simulink model "TrayectoriaReal"  (R2018a)
settings: Solver=ode45  StartTime=0.0  StopTime=Tfin2  RelTol=1e-3  EnableMultiTasking=on
values from neighbouring files (symbols this model uses):
  dyn = [dh dyn]    [trabajoRob.m]
  dyne = (ones(6,20)+err).*dyn    [trabajoRob.m]
  g = [0 0 -9.81]    [trabajoRob.m]
  Qt2 = [[1:length(Qt2)]'*Ts2,Qt2]    [trabajoRob.m]    (also in trayectoria.m = [[0:length(trayq)-1]'*Ts2 trayq])
  Tfin = 25    [trabajoRob.m]
  Ts = Tfin/(puntos-1)    (= 0.0501002004008)    [trabajoRob.m]
  Ts2 = 0.01    [trabajoRob.m]    (also in trayectoria.m)
libraries: HEMERO x2, peGeneralControl x2
settings Model: ExtModeTrigMode=oneshot  ExtModeArmWhenConnect=off  Creator=Pablo Linares  LastModifiedBy=Pablo Linares
settings DataIOCC: SaveFormat=Array  SignalLoggingSaveFormat=ModelDataLogs
settings OptimizationCC: BlockReduction=off  BooleanDataType=off
settings DebuggingCC: SaveWithParameterizedLinksMsg=none  UnderspecifiedInitializationDetection=Classic  MergeDetectMultiDrivingBlocksExec=none  SignalResolutionControl=TryResolveAllWithWarning  MultiTaskDSMMsg=warning  MultiTaskCondExecSysMsg=none
settings HardwareCC: TargetUnknown=on
settings ModelReferenceCC: PropagateSignalLabelsOutOfModel=off
settings GRTTargetCC: TargetLangStandard=C89/C90 (ANSI)  CombineOutputUpdateFcns=off  GRTInterface=on

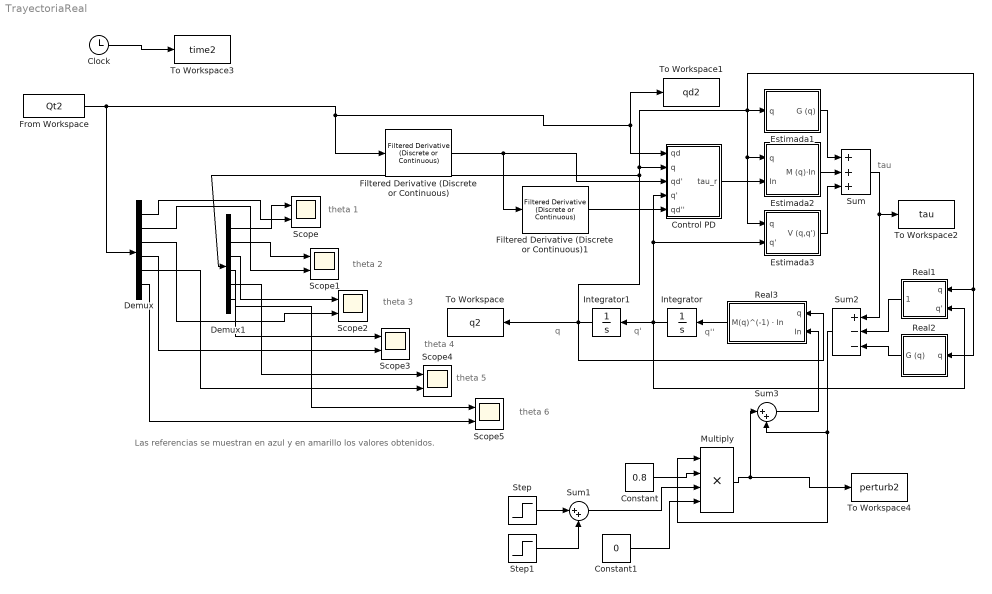
== system TrayectoriaReal ==
  note: Las referencias se muestran en azul y en amarillo los valores obtenidos.
  note: theta 6
  note: theta 5
  note: theta 4
  note: theta 3
  note: theta 2
  note: theta 1
  note: tau
  note: q
  note: q'
  note: q''
  Clock : Clock
  Constant : Constant  Value=0.8
  Constant1 : Constant  Value=0
  Control PD : Subsystem  mask(Controlador PD){Kp=[1 0 0 0 0 0;0 1 0 0 0 0; 0 0 1 0 0 0; 0 0 0 1 0 0; 0 0 0 0 1 0; 0 0 0 0 0 1]*986.96, Kv=[1 0 0 0 0 0;0 1 0 0 0 0; 0 0 1 0 0 0; 0 0 0 1 0 0; 0 0 0 0 1 0; 0 0 0 0 0 1]*62.83}
      mask prompts: Kp "Introduzca la matriz Kp:"; Kv "Introduzca la matriz Kv:"
      mask help: Calcula el par tau_r correspondiente a la técnica del par computado usando un controlador PD.
  Demux : Demux  Outputs=6
  Demux1 : Demux  Outputs=6
  Estimada1 : Subsystem  mask(Término gravitatorio){dyn=dyne, grav=g}
      mask prompts: dyn "Matriz de parámetros cinemáticos y dinámicos:"; grav "Vector aceleración de la gravedad:"
      mask help: Este bloque calcula el par correspondiente al término gravitatorio.
  Estimada2 : Subsystem  mask(Término asociado a la matriz de masas){dyn=dyne}
      mask prompts: dyn "Matriz de parámetros cinemáticos y dinámicos:"
      mask help: Este bloque calcula el par correspondiente al término en el que aparece la matriz de masas.
  Estimada3 : Subsystem  mask(Términos centrífugos y de Coriolis){dyn=dyne}
      mask prompts: dyn "Matriz de parámetros cinemáticos y dinámicos:"
      mask help: Este bloque calcula el par correspondiente a los términos centrífugos y de Coriolis.
  Filtered Derivative (Discrete or Continuous) : peGeneralControl/Filtered Derivative (Discrete or Continuous)  K=1  T=0.01  B=inf  A=-inf  minRatio=10  Ts=Ts
  Filtered Derivative (Discrete or Continuous)1 : peGeneralControl/Filtered Derivative (Discrete or Continuous)  K=1  T=0.01  B=inf  A=-inf  minRatio=10  Ts=Ts
  From Workspace : FromWorkspace  VariableName=Qt2  SampleTime=Ts2
  Integrator : Integrator  InitialCondition=[0;0;0;0;0;0]
  Integrator1 : Integrator  InitialCondition=Qt2(1,2:7)'
  Multiply : Product  Inputs=4
  Real1 : Subsystem  mask(Términos centrífugos y de Coriolis){dyn=dyn}
      mask prompts: dyn "Matriz de parámetros cinemáticos y dinámicos:"
      mask help: Este bloque calcula el par correspondiente a los términos centrífugos y de Coriolis.
  Real2 : Subsystem  mask(Término gravitatorio){dyn=dyn, grav=g}
      mask prompts: dyn "Matriz de parámetros cinemáticos y dinámicos:"; grav "Vector aceleración de la gravedad:"
      mask help: Este bloque calcula el par correspondiente al término gravitatorio.
  Real3 : Subsystem  mask(Inversa de la matriz de masas){dyn=dyn}
      mask prompts: dyn "Matriz de parámetros cinemáticos y dinámicos:"
      mask help: Este bloque calcula el producto de la inversa de la matriz de masas por el vector columna In que se le pasa como entrada.
  Scope{,1..5} (6 alike) : Scope  NumInputPorts=2
  Step : Step  Time=Tfin*0.5  SampleTime=0
  Step1 : Step  Time=Tfin*0.6  After=-1  SampleTime=0
  Sum : Sum  Inputs=+++  SaturateOnIntegerOverflow=on  InputSameDT=on  OutDataTypeStr=Inherit: Same as first input
  Sum1 : Sum  Inputs=|++
  Sum2 : Sum  Inputs=+--  SaturateOnIntegerOverflow=on  InputSameDT=on  OutDataTypeStr=Inherit: Same as first input
  Sum3 : Sum  Inputs=|++
  To Workspace : ToWorkspace  VariableName=q2  SampleTime=Ts2
  To Workspace1 : ToWorkspace  VariableName=qd2  SampleTime=Ts2
  To Workspace2 : ToWorkspace  VariableName=tau  SampleTime=-1
  To Workspace3 : ToWorkspace  VariableName=time2  SampleTime=Ts2
      settings: Save2DSignal=2-D array (concatenate along first dimension)
  To Workspace4 : ToWorkspace  VariableName=perturb2  SampleTime=Ts2
  wires:
  Sum/1 -> To Workspace2/1, Sum2/1
  Control PD/1(tau_r) -> Estimada2/2(In)
  Estimada2/1(M (q)·In) -> Sum/2
  Estimada1/1(G (q)) -> Sum/1
  Estimada3/1(V (q,q')) -> Sum/3
  Real2/1(G (q)) -> Sum2/3
  Real1/1(V (q,q')) -> Sum2/2
  Integrator/1 -> Integrator1/1, Control PD/4(q'), Estimada3/2(q'), Real1/2(q')
  Integrator1/1 -> Estimada1/1(q), Estimada2/1(q), Estimada3/1(q), Real1/1(q), Real2/1(q), Control PD/2(q), Demux1/1, To Workspace/1, Real3/1(q)
  Real3/1(M(q)^(-1) · In) -> Integrator/1
  Filtered Derivative (Discrete or Continuous)/1 -> Filtered Derivative (Discrete or Continuous)1/1, Control PD/3(qd')
  Filtered Derivative (Discrete or Continuous)1/1 -> Control PD/5(qd'')
  Demux1/2 -> Scope1/1
  Demux/2 -> Scope1/2
  Demux1/3 -> Scope2/1
  Demux/3 -> Scope2/2
  Demux1/4 -> Scope3/1
  Demux/4 -> Scope3/2
  Demux1/5 -> Scope4/1
  Demux/5 -> Scope4/2
  Demux1/6 -> Scope5/1
  Demux/6 -> Scope5/2
  From Workspace/1 -> Filtered Derivative (Discrete or Continuous)/1, To Workspace1/1, Control PD/1(qd), Demux/1
  Demux1/1 -> Scope/1
  Demux/1 -> Scope/2
  Clock/1 -> To Workspace3/1
  Constant/1 -> Multiply/2
  Step/1 -> Sum1/1
  Step1/1 -> Sum1/2
  Sum1/1 -> Multiply/3
  Multiply/1 -> Sum3/1, To Workspace4/1
  Sum2/1 -> Sum3/2, Multiply/1
  Sum3/1 -> Real3/2(In)
  Constant1/1 -> Multiply/4

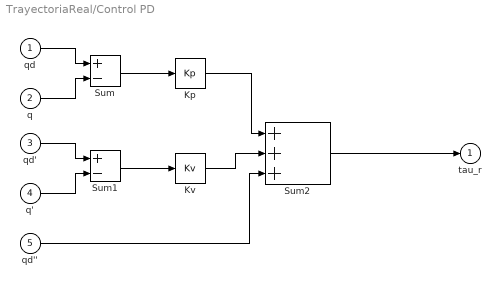
== system TrayectoriaReal/Control PD ==
  qd : Inport
  q : Inport  Port=2
  qd' : Inport  Port=3
  q' : Inport  Port=4
  qd'' : Inport  Port=5
  Kp : HEMERO/Robots manipuladores base fija/Control basado en el modelo/Par Computado/Ejemplos/Ejemplo H.5.2/Control PD/Kp  K=Kp
  Kv : HEMERO/Robots manipuladores base fija/Control basado en el modelo/Par Computado/Ejemplos/Ejemplo H.5.2/Control PD/Kv  K=Kv
  Sum : Sum  Inputs=+-  SaturateOnIntegerOverflow=on  InputSameDT=on  OutDataTypeStr=Inherit: Same as first input
  Sum1 : Sum  Inputs=+-  SaturateOnIntegerOverflow=on  InputSameDT=on  OutDataTypeStr=Inherit: Same as first input
  Sum2 : Sum  Inputs=+++  SaturateOnIntegerOverflow=on  InputSameDT=on  OutDataTypeStr=Inherit: Same as first input
  tau_r : Outport  InitialOutput=0
  wires:
  qd/1 -> Sum/1
  q/1 -> Sum/2
  qd'/1 -> Sum1/1
  q'/1 -> Sum1/2
  Sum/1 -> Kp/1
  Sum1/1 -> Kv/1
  Kv/1 -> Sum2/2
  Kp/1 -> Sum2/1
  qd''/1 -> Sum2/3
  Sum2/1 -> tau_r/1

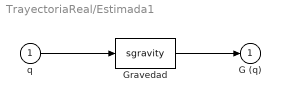
== system TrayectoriaReal/Estimada1 ==
  q : Inport
  Gravedad : S-Function  FunctionName=sgravity  Parameters=dyn,grav  SFunctionDeploymentMode=off  EnableBusSupport=off
  G (q) : Outport  InitialOutput=0
  wires:
  q/1 -> Gravedad/1
  Gravedad/1 -> G (q)/1

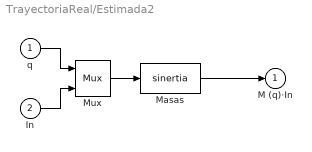
== system TrayectoriaReal/Estimada2 ==
  q : Inport
  In : Inport  Port=2
  Masas : S-Function  FunctionName=sinertia  Parameters=dyn  SFunctionDeploymentMode=off  EnableBusSupport=off
  Mux : Mux  Inputs=2
  M (q)·In : Outport  InitialOutput=0
  wires:
  Mux/1 -> Masas/1
  q/1 -> Mux/1
  In/1 -> Mux/2
  Masas/1 -> M (q)·In/1

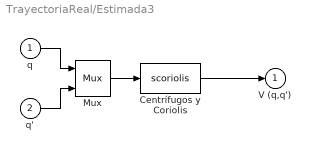
== system TrayectoriaReal/Estimada3 ==
  q : Inport
  q' : Inport  Port=2
  Centrífugos y Coriolis : S-Function  FunctionName=scoriolis  Parameters=dyn  SFunctionDeploymentMode=off  EnableBusSupport=off
  Mux : Mux  Inputs=2
  V (q,q') : Outport  InitialOutput=0
  wires:
  Mux/1 -> Centrífugos y Coriolis/1
  q/1 -> Mux/1
  q'/1 -> Mux/2
  Centrífugos y Coriolis/1 -> V (q,q')/1

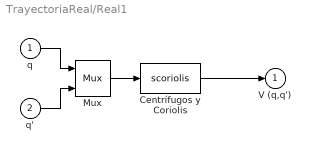
== system TrayectoriaReal/Real1 ==
  q : Inport
  q' : Inport  Port=2
  Centrífugos y Coriolis : S-Function  FunctionName=scoriolis  Parameters=dyn  SFunctionDeploymentMode=off  EnableBusSupport=off
  Mux : Mux  Inputs=2
  V (q,q') : Outport  InitialOutput=0
  wires:
  Mux/1 -> Centrífugos y Coriolis/1
  q/1 -> Mux/1
  q'/1 -> Mux/2
  Centrífugos y Coriolis/1 -> V (q,q')/1

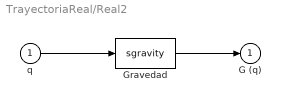
== system TrayectoriaReal/Real2 ==
  q : Inport
  Gravedad : S-Function  FunctionName=sgravity  Parameters=dyn,grav  SFunctionDeploymentMode=off  EnableBusSupport=off
  G (q) : Outport  InitialOutput=0
  wires:
  q/1 -> Gravedad/1
  Gravedad/1 -> G (q)/1

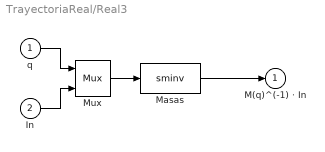
== system TrayectoriaReal/Real3 ==
  q : Inport
  In : Inport  Port=2
  Masas : S-Function  FunctionName=sminv  Parameters=dyn  SFunctionDeploymentMode=off  EnableBusSupport=off
  Mux : Mux  Inputs=2
  M(q)^(-1) · In : Outport  InitialOutput=0
  wires:
  Mux/1 -> Masas/1
  q/1 -> Mux/1
  In/1 -> Mux/2
  Masas/1 -> M(q)^(-1) · In/1
